simulink library "SpeakerSubsystemLibrary_1_0_0"  (R2022b)
settings: Solver=VariableStepAuto  StartTime=0.0  StopTime=10.0  RelTol=1e-3
undefined symbols (not defined in the file): BL_0, BL_1, BL_2, BL_3, BL_4, D_0, D_1, D_2, D_3, D_4, K_0, K_1, K_2, K_3, K_4, L2, Le_0, Le_1, Le_2, Le_3, Le_4, Mm, R2, Re, Sd
libraries: fl_lib x15, acoustical_lib x6
settings Model: Creator=stephenthompson  LastModifiedBy=sct12
settings ModelReferenceCC: EnableRefExpFcnMdlSchedulingChecks=on

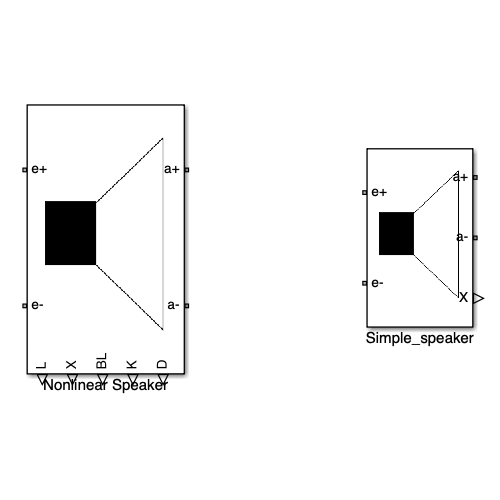
[thumbnail: Simulink's stored preview of the top-level diagram]
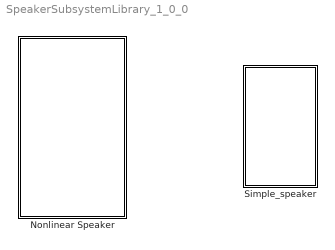
== system SpeakerSubsystemLibrary_1_0_0 ==
  Nonlinear Speaker : Subsystem  mask{Sd=Sd, Sd_unit=cm^2, Sd_conf=compiletime, mass=Mm, mass_unit=g, mass_conf=compiletime, R=Re, R_unit=Ohm, R_conf=compiletime, L2=L2, L2_unit=H, L2_conf=compiletime, R2=R2, R2_unit=Ohm, R2_conf=compiletime, L0_of_x=Le_0, L0_of_x_unit=H, L0_of_x_conf=compiletime, L1_of_x=Le_1, L1_of_x_unit=H/m, L1_of_x_conf=compiletime, L2_of_x=Le_2, L2_of_x_unit=H/m^2, L2_of_x_conf=compiletime, L3_of_x=Le_3, L3_of_x_unit=H/m^3, L3_of_x_conf=compiletime, L4_of_x=Le_4, L4_of_x_unit=H/m^4, L4_of_x_conf=compiletime, Bl0=BL_0, Bl0_unit=N/A, Bl0_conf=compiletime, Bl1=BL_1, Bl1_unit=N/(A*m), Bl1_conf=compiletime, Bl2=BL_2, Bl2_unit=N/(A*m^2), Bl2_conf=compiletime, Bl3=BL_3, Bl3_unit=N/(A*m^3), Bl3_conf=compiletime, Bl4=BL_4, Bl4_unit=N/(A*m^4), Bl4_conf=compiletime, K0=K_0, K0_unit=N/m, K0_conf=compiletime, K1=K_1, K1_unit=N/m^2, K1_conf=compiletime, K2=K_2, K2_unit=N/m^3, K2_conf=compiletime, K3=K_3, K3_unit=N/m^4, K3_conf=compiletime, K4=K_4, K4_unit=N/m^5, K4_conf=compiletime, D0=D_0, D0_unit=N*s/m, D0_conf=compiletime, D1=D_1, D1_unit=N*s^2/m^2, D1_conf=compiletime, D2=D_2, D2_unit=N*s^3/m^3, D2_conf=compiletime, D3=D_3, D3_unit=N*s^4/m^4, D3_conf=compiletime, D4=D_4, D4_unit=N*s^5/m^5, D4_conf=compiletime}
      mask prompts: Sd "Cone Area Sd"; mass "Moving Mass"; R "Coil Resistance"; Bl0 "Constant part in force factor"; Bl1 "1st order coefficient"; Bl2 "2nd order coefficient"; Bl3 "3rd order coefficient"; Bl4 "4th order coefficient"; K0 "constant part in stiffness"; K1 "1st order coefficient"; K2 "2nd order coefficient"; K3 "3rd order coefficient"; K4 "4th order coefficient"; D0 "constant part in stiffness"; D1 "N1st order coefficient"; D2 "N2nd order coefficient"; D3 "3rd order coefficient"; D4 "N*4th order coefficient"
      settings: PortSchema="{\"entries\":[{\"content\":{\"sides\":[{\"content\":{\"connectorIds\":[\"LConn1\",\"LConn2\"]},\"type\":\"ConnectorPlacement.EquallySpacedRectSide\",\"uuid\":\"f64a30bf-56c6-47b5-b4bc-71101fcbb95a\"},{\"content\":{\"connectorIds\":[\"RConn1\",\"RConn2\"],\"side\":\"RIGHT\"},\"type\":\"ConnectorPlacement.EquallySpacedRectSide\",\"uuid\":\"026264a5-a5ab-4ec3-912f-977c3d8fe047\"},{\"content\":{\"connectorIds\":[],\"side\":\"TOP\"},\"type\":\"ConnectorPlacement.EquallySpacedRectSide\",\"uuid\":\"73a10c58-d118-4274-a8f1-6138ac105e53\"},{\"content\":{\"connectorIds\":[\"RConn3\",\"RConn4\",\"RConn5\",\"RConn6\",\"RConn7\"],\"side\":\"BOTTOM\"},\"type\":\"ConnectorPlacement.EquallySpacedRectSide\",\"uuid\":\"493ec49a-e47d-475d-ab4f-1f36cc0e6d29\"}]},\"type\":\"ConnectorPlacement.EquallySpacedConnector\",\"uuid\":\"07e5b91c-fb95-4bee-828a-833440d87f91\"}],\"packageUris\":[\"http://schema.mathworks.com/mf0/Connector/R2020b\"],\"version\":\"1.0\"}"
      mask TypeOptions Sd: Area_xfrm/Sd
      mask TypeOptions Sd_unit: Area_xfrm/Sd_unit
      mask TypeOptions Sd_conf: Area_xfrm/Sd_conf
      mask TypeOptions mass: Mm/mass
      mask TypeOptions mass_unit: Mm/mass_unit
      mask TypeOptions mass_conf: Mm/mass_conf
      mask TypeOptions R: Re/R
      mask TypeOptions R_unit: Re/R_unit
      mask TypeOptions R_conf: Re/R_conf
      mask TypeOptions L2: L2/l
      mask TypeOptions L2_unit: L2/l_unit
      mask TypeOptions L2_conf: L2/l_conf
      mask TypeOptions R2: R2/R
      mask TypeOptions R2_unit: R2/R_unit
      mask TypeOptions R2_conf: R2/R_conf
      mask TypeOptions L0_of_x: Le_of_x/L0
      mask TypeOptions L0_of_x_unit: Le_of_x/L0_unit
      mask TypeOptions L0_of_x_conf: Le_of_x/L0_conf
      mask TypeOptions L1_of_x: Le_of_x/L1
      mask TypeOptions L1_of_x_unit: Le_of_x/L1_unit
      mask TypeOptions L1_of_x_conf: Le_of_x/L1_conf
      mask TypeOptions L2_of_x: Le_of_x/L2
      mask TypeOptions L2_of_x_unit: Le_of_x/L2_unit
      mask TypeOptions L2_of_x_conf: Le_of_x/L2_conf
      mask TypeOptions L3_of_x: Le_of_x/L3
      mask TypeOptions L3_of_x_unit: Le_of_x/L3_unit
      mask TypeOptions L3_of_x_conf: Le_of_x/L3_conf
      mask TypeOptions L4_of_x: Le_of_x/L4
      mask TypeOptions L4_of_x_unit: Le_of_x/L4_unit
      mask TypeOptions L4_of_x_conf: Le_of_x/L4_conf
      mask TypeOptions Bl0: BL_of_x/Bl0
      mask TypeOptions Bl0_unit: BL_of_x/Bl0_unit
      mask TypeOptions Bl0_conf: BL_of_x/Bl0_conf
      mask TypeOptions Bl1: BL_of_x/Bl1
      mask TypeOptions Bl1_unit: BL_of_x/Bl1_unit
      mask TypeOptions Bl1_conf: BL_of_x/Bl1_conf
      mask TypeOptions Bl2: BL_of_x/Bl2
      mask TypeOptions Bl2_unit: BL_of_x/Bl2_unit
      mask TypeOptions Bl2_conf: BL_of_x/Bl2_conf
      mask TypeOptions Bl3: BL_of_x/Bl3
      mask TypeOptions Bl3_unit: BL_of_x/Bl3_unit
      mask TypeOptions Bl3_conf: BL_of_x/Bl3_conf
      mask TypeOptions Bl4: BL_of_x/Bl4
      mask TypeOptions Bl4_unit: BL_of_x/Bl4_unit
      mask TypeOptions Bl4_conf: BL_of_x/Bl4_conf
      mask TypeOptions K0: K_of_x/K0
      mask TypeOptions K0_unit: K_of_x/K0_unit
      mask TypeOptions K0_conf: K_of_x/K0_conf
      mask TypeOptions K1: K_of_x/K1
      mask TypeOptions K1_unit: K_of_x/K1_unit
      mask TypeOptions K1_conf: K_of_x/K1_conf
      mask TypeOptions K2: K_of_x/K2
      mask TypeOptions K2_unit: K_of_x/K2_unit
      mask TypeOptions K2_conf: K_of_x/K2_conf
      mask TypeOptions K3: K_of_x/K3
      mask TypeOptions K3_unit: K_of_x/K3_unit
      mask TypeOptions K3_conf: K_of_x/K3_conf
      mask TypeOptions K4: K_of_x/K4
      mask TypeOptions K4_unit: K_of_x/K4_unit
      mask TypeOptions K4_conf: K_of_x/K4_conf
      mask TypeOptions D0: Rm_of_v/D0
      mask TypeOptions D0_unit: Rm_of_v/D0_unit
      mask TypeOptions D0_conf: Rm_of_v/D0_conf
      mask TypeOptions D1: Rm_of_v/D1
      mask TypeOptions D1_unit: Rm_of_v/D1_unit
      mask TypeOptions D1_conf: Rm_of_v/D1_conf
      mask TypeOptions D2: Rm_of_v/D2
      mask TypeOptions D2_unit: Rm_of_v/D2_unit
      mask TypeOptions D2_conf: Rm_of_v/D2_conf
      mask TypeOptions D3: Rm_of_v/D3
      mask TypeOptions D3_unit: Rm_of_v/D3_unit
      mask TypeOptions D3_conf: Rm_of_v/D3_conf
      mask TypeOptions D4: Rm_of_v/D4
      mask TypeOptions D4_unit: Rm_of_v/D4_unit
      mask TypeOptions D4_conf: Rm_of_v/D4_conf
      mask DialogControl Container4 Prompt: Inductor Parameters
      mask DialogControl Container5 Prompt: Force Factor BL Parameters
      mask DialogControl Container6 Prompt: Spring Stiffness Parameters
      mask DialogControl Container7 Prompt: Mechanical Damping Parameters
      mask Display: image('$imagefile'); % Use "Edit Image" on toolstrip to change.
  Simple_speaker : Subsystem  mask{Re=7.8, Re_unit=Ohm, Re_conf=compiletime, Le=0.124, Le_unit=H, Le_conf=compiletime, L2=1e-6, L2_unit=H, L2_conf=compiletime, R2=1, R2_unit=Ohm, R2_conf=compiletime, BL=5.63, BL_unit=V*s/m, BL_conf=compiletime, Mm=4.8, Mm_unit=g, Mm_conf=compiletime, K=1/1.05e-3, K_unit=N/m, K_conf=compiletime, D=1, D_unit=N*s/m, D_conf=compiletime, Sd=30.4, Sd_unit=cm^2, Sd_conf=compiletime}
      mask prompts: Re "Coil Resistance"; Le "Coil Inductance"; BL "Force Factor BL"; Mm "Cone Moving Mass"; K "Cone Mounting Stiffness"; D "Mechanical Resistance"; Sd "Cone Area"
      mask TypeOptions Re: Re/R
      mask TypeOptions Re_unit: Re/R_unit
      mask TypeOptions Re_conf: Re/R_conf
      mask TypeOptions Le: Le/l
      mask TypeOptions Le_unit: Le/l_unit
      mask TypeOptions Le_conf: Le/l_conf
      mask TypeOptions L2: L2/l
      mask TypeOptions L2_unit: L2/l_unit
      mask TypeOptions L2_conf: L2/l_conf
      mask TypeOptions R2: R2/R
      mask TypeOptions R2_unit: R2/R_unit
      mask TypeOptions R2_conf: R2/R_conf
      mask TypeOptions BL: BL/K
      mask TypeOptions BL_unit: BL/K_unit
      mask TypeOptions BL_conf: BL/K_conf
      mask TypeOptions Mm: Mm/mass
      mask TypeOptions Mm_unit: Mm/mass_unit
      mask TypeOptions Mm_conf: Mm/mass_conf
      mask TypeOptions K: K/spr_rate
      mask TypeOptions K_unit: K/spr_rate_unit
      mask TypeOptions K_conf: K/spr_rate_conf
      mask TypeOptions D: D/D
      mask TypeOptions D_unit: D/D_unit
      mask TypeOptions D_conf: D/D_conf
      mask TypeOptions Sd: Sd/Sd
      mask TypeOptions Sd_unit: Sd/Sd_unit
      mask TypeOptions Sd_conf: Sd/Sd_conf
      mask Display: image('$imagefile'); % Use "Edit Image" on toolstrip to change.

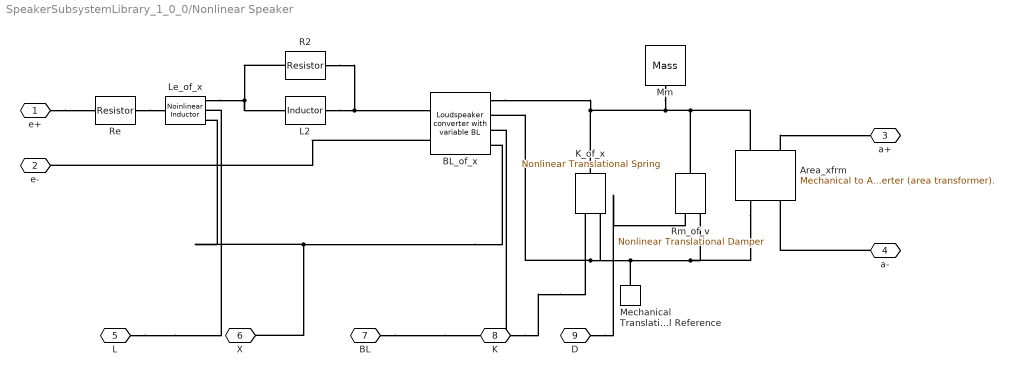
== system SpeakerSubsystemLibrary_1_0_0/Nonlinear Speaker ==
  Area_xfrm : acoustical_lib/Acoustical Elements/Mechanical to Acoustical Converter (area transformer).  Sd=Sd cm^2  u_specify=off  u_priority=None  u=0 m^3/s  u_nominal_specify=off  u_nominal_unit=m^3/s  u_nominal_value=1  p_specify=off  p_priority=None  p=0 Pa  p_nominal_specify=off  p_nominal_unit=Pa  p_nominal_value=1  f_specify=off  f_priority=None  f=0 N  f_nominal_specify=off  f_nominal_unit=N  f_nominal_value=1  v_specify=off  v_priority=None  v=0 m/s  v_nominal_specify=off  v_nominal_unit=m/s  v_nominal_value=1
      settings: SourceProductName=Acoustical  InternalSimscapePortConfiguration="{\"Bottom\":[],\"Left\":[{\"id\":\"pp\",\"label\":\"+\",\"type\":\"acoustical.acoustical\"},{\"id\":\"R\",\"label\":\"R\",\"type\":\"foundation.mechanical.translational.translational\"}],\"Right\":[{\"id\":\"nn\",\"label\":\"-\",\"type\":\"acoustical.acoustical\"},{\"id\":\"C\",\"label\":\"C\",\"type\":\"foundation.mechanical.translational.translational\"}],\"Top\":[]}"
  BL_of_x : acoustical_lib/Moving Coil Speakers/speaker_nonlinear_blocks/Loudspeaker converter with variable BL  Bl0=Bl0 N/A  Bl1=Bl1 N/(A*m)  Bl2=Bl2 N/(A*m^2)  Bl3=Bl3 N/(A*m^3)  Bl4=Bl4 N/(A*m^4)  i_specify=off  i_priority=None  i=0 A  i_nominal_specify=off  i_nominal_unit=A  i_nominal_value=1  v_specify=off  v_priority=None  v=0 V  v_nominal_specify=off  v_nominal_unit=V  v_nominal_value=1  f_specify=off  f_priority=None  f=0 N  f_nominal_specify=off  f_nominal_unit=N  f_nominal_value=1  u_specify=off  u_priority=None  u=0 m/s  u_nominal_specify=off  u_nominal_unit=m/s  u_nominal_value=1
      settings: SourceProductName=Acoustical  InternalSimscapePortConfiguration="{\"Bottom\":[{\"id\":\"BL\",\"label\":\"BL\",\"type\":\"output\"},{\"id\":\"X\",\"label\":\"\",\"type\":\"output\"}],\"Left\":[{\"id\":\"p\",\"label\":\"+\",\"type\":\"foundation.electrical.electrical\"},{\"id\":\"n\",\"label\":\"-\",\"type\":\"foundation.electrical.electrical\"}],\"Right\":[{\"id\":\"R\",\"label\":\"R\",\"type\":\"foundation.mechanical.translational.translational\"},{\"id\":\"C\",\"label\":\"C\",\"type\":\"foundation.mechanical.translational.translational\"}],\"Top\":[]}"
  K_of_x : acoustical_lib/Moving Coil Speakers/speaker_nonlinear_blocks/Nonlinear Translational Spring  K0=K0 N/m  K1=K1 N/m^2  K2=K2 N/m^3  K3=K3 N/m^4  K4=K4 N/m^5  v_specify=off  v_priority=None  v=0 m/s  v_nominal_specify=off  v_nominal_unit=m/s  v_nominal_value=1  f_specify=off  f_priority=None  f=0 N  f_nominal_specify=off  f_nominal_unit=N  f_nominal_value=1  x_specify=off  x_priority=High  x=0 m  x_nominal_specify=off  x_nominal_unit=m  x_nominal_value=1
      settings: SourceProductName=Acoustical  InternalSimscapePortConfiguration="{\"Bottom\":[{\"id\":\"K\",\"label\":\"K\",\"type\":\"output\"}],\"Left\":[{\"id\":\"R\",\"label\":\"R\",\"type\":\"foundation.mechanical.translational.translational\"}],\"Right\":[{\"id\":\"C\",\"label\":\"C\",\"type\":\"foundation.mechanical.translational.translational\"}],\"Top\":[]}"
  L2 : fl_lib/Electrical/Electrical Elements/Inductor  l=L2 H  r=0 Ohm  g=1e-9 1/Ohm  i_specify=off  i_priority=None  i=0 A  i_nominal_specify=off  i_nominal_unit=A  i_nominal_value=1  v_specify=off  v_priority=None  v=0 V  v_nominal_specify=off  v_nominal_unit=V  v_nominal_value=1  i_L_specify=off  i_L_priority=High  i_L=0 A  i_L_nominal_specify=off  i_L_nominal_unit=A  i_L_nominal_value=1
  Le_of_x : acoustical_lib/Moving Coil Speakers/speaker_nonlinear_blocks/Noinlinear Inductor  r=0 Ohm  g=1e-9 1/Ohm  L0=L0_of_x H  L1=L1_of_x H/m  L2=L2_of_x H/m^2  L3=L3_of_x H/m^3  L4=L4_of_x H/m^4  i_specify=off  i_priority=None  i=0 A  i_nominal_specify=off  i_nominal_unit=A  i_nominal_value=1  v_specify=off  v_priority=None  v=0 V  v_nominal_specify=off  v_nominal_unit=V  v_nominal_value=1  i_L_specify=off  i_L_priority=High  i_L=0 A  i_L_nominal_specify=off  i_L_nominal_unit=A  i_L_nominal_value=1
      settings: SourceProductName=Acoustical  InternalSimscapePortConfiguration="{\"Bottom\":[{\"id\":\"L\",\"label\":\"L\",\"type\":\"output\"},{\"id\":\"X\",\"label\":\"x\",\"type\":\"input\"}],\"Left\":[{\"id\":\"p\",\"label\":\"+\",\"type\":\"foundation.electrical.electrical\"}],\"Right\":[{\"id\":\"n\",\"label\":\"-\",\"type\":\"foundation.electrical.electrical\"}],\"Top\":[]}"
  Mechanical Translational Reference : fl_lib/Mechanical/Translational Elements/Mechanical Translational Reference
  Mm : fl_lib/Mechanical/Translational Elements/Mass  mass=mass g  num_ports=foundation.enum.numPorts2.one  v_specify=off  v_priority=High  v=0 m/s  v_nominal_specify=off  v_nominal_unit=m/s  v_nominal_value=1  f_specify=off  f_priority=None  f=0 N  f_nominal_specify=off  f_nominal_unit=N  f_nominal_value=1
  R2 : fl_lib/Electrical/Electrical Elements/Resistor  R=R2 Ohm  i_specify=off  i_priority=None  i=0 A  i_nominal_specify=off  i_nominal_unit=A  i_nominal_value=1  v_specify=off  v_priority=None  v=0 V  v_nominal_specify=off  v_nominal_unit=V  v_nominal_value=1
  Re : fl_lib/Electrical/Electrical Elements/Resistor  R=R Ohm  i_specify=off  i_priority=None  i=0 A  i_nominal_specify=off  i_nominal_unit=A  i_nominal_value=1  v_specify=off  v_priority=None  v=0 V  v_nominal_specify=off  v_nominal_unit=V  v_nominal_value=1
  Rm_of_v : acoustical_lib/Moving Coil Speakers/speaker_nonlinear_blocks/Nonlinear Translational Damper  D0=D0 N*s/m  D1=D1 N*s^2/m^2  D2=D2 N*s^3/m^3  D3=D3 N*s^4/m^4  D4=D4 N*s^5/m^5  v_specify=off  v_priority=None  v=0 m/s  v_nominal_specify=off  v_nominal_unit=m/s  v_nominal_value=1  f_specify=off  f_priority=None  f=0 N  f_nominal_specify=off  f_nominal_unit=N  f_nominal_value=1  x_specify=off  x_priority=High  x=0 m  x_nominal_specify=off  x_nominal_unit=m  x_nominal_value=1
      settings: SourceProductName=Acoustical  InternalSimscapePortConfiguration="{\"Bottom\":[{\"id\":\"D\",\"label\":\"D\",\"type\":\"output\"}],\"Left\":[{\"id\":\"R\",\"label\":\"R\",\"type\":\"foundation.mechanical.translational.translational\"}],\"Right\":[{\"id\":\"C\",\"label\":\"C\",\"type\":\"foundation.mechanical.translational.translational\"}],\"Top\":[]}"
  e+ : PMIOPort  Side=Left
  e- : PMIOPort  Port=2  Side=Left
  a+ : PMIOPort  Port=3  Side=Right
  a- : PMIOPort  Port=4  Side=Right
  L : PMIOPort  Port=5  Side=Right
  X : PMIOPort  Port=6  Side=Right
  BL : PMIOPort  Port=7  Side=Right
  K : PMIOPort  Port=8  Side=Right
  D : PMIOPort  Port=9  Side=Right
  connections:
  X/RConn1 -- BL_of_x/RConn4 -- Le_of_x/RConn3
  e+/RConn1 -- Re/LConn1
  Rm_of_v/LConn1 -- Area_xfrm/LConn2 -- Mm/LConn1 -- K_of_x/LConn1 -- BL_of_x/RConn1
  Re/RConn1 -- Le_of_x/LConn1
  Area_xfrm/LConn1 -- a+/RConn1
  D/RConn1 -- Rm_of_v/RConn2
  BL_of_x/LConn2 -- e-/RConn1
  Area_xfrm/RConn2 -- Mechanical Translational Reference/LConn1 -- BL_of_x/RConn2 -- K_of_x/RConn1 -- Rm_of_v/RConn1
  L/RConn1 -- Le_of_x/RConn2
  BL/RConn1 -- BL_of_x/RConn3
  K/RConn1 -- K_of_x/RConn2
  a-/RConn1 -- Area_xfrm/RConn1
  Le_of_x/RConn1 -- R2/LConn1 -- L2/LConn1
  L2/RConn1 -- R2/RConn1 -- BL_of_x/LConn1

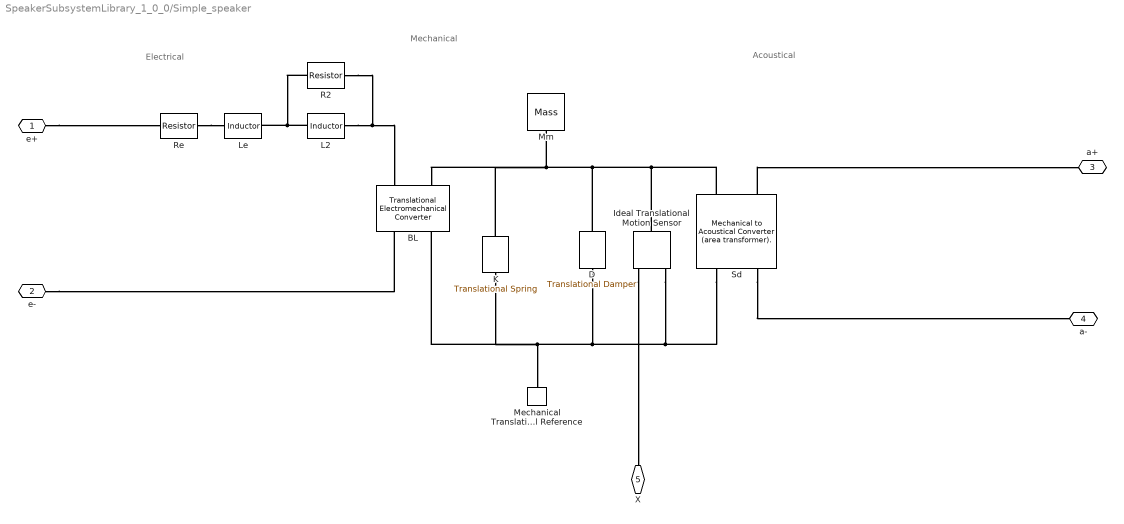
== system SpeakerSubsystemLibrary_1_0_0/Simple_speaker ==
  note: Acoustical
  note: Mechanical
  note: Electrical
  BL : fl_lib/Electrical/Electrical Elements/Translational Electromechanical Converter  K=BL V*s/m  i_specify=off  i_priority=None  i=0 A  i_nominal_specify=off  i_nominal_unit=A  i_nominal_value=1  v_specify=off  v_priority=None  v=0 V  v_nominal_specify=off  v_nominal_unit=V  v_nominal_value=1  f_specify=off  f_priority=None  f=0 N  f_nominal_specify=off  f_nominal_unit=N  f_nominal_value=1  u_specify=off  u_priority=None  u=0 m/s  u_nominal_specify=off  u_nominal_unit=m/s  u_nominal_value=1
      settings: InternalSimscapePortConfiguration="{\"Bottom\":[],\"Left\":[{\"id\":\"p\",\"label\":\"+\",\"type\":\"foundation.electrical.electrical\"},{\"id\":\"R\",\"label\":\"R\",\"type\":\"foundation.mechanical.translational.translational\"}],\"Right\":[{\"id\":\"n\",\"label\":\"-\",\"type\":\"foundation.electrical.electrical\"},{\"id\":\"C\",\"label\":\"C\",\"type\":\"foundation.mechanical.translational.translational\"}],\"Top\":[]}"
  D : fl_lib/Mechanical/Translational Elements/Translational Damper  D=D N*s/m  v_specify=off  v_priority=None  v=0 m/s  v_nominal_specify=off  v_nominal_unit=m/s  v_nominal_value=1  f_specify=off  f_priority=None  f=0 N  f_nominal_specify=off  f_nominal_unit=N  f_nominal_value=1
  Ideal Translational Motion Sensor : fl_lib/Mechanical/Mechanical Sensors/Ideal Translational Motion Sensor  reference=foundation.enum.MeasurementReference.difference  acceleration_port=false  velocity_port=true  position_port=true  offset=0 m
  K : fl_lib/Mechanical/Translational Elements/Translational Spring  spr_rate=K N/m  v_specify=off  v_priority=None  v=0 m/s  v_nominal_specify=off  v_nominal_unit=m/s  v_nominal_value=1  f_specify=off  f_priority=None  f=0 N  f_nominal_specify=off  f_nominal_unit=N  f_nominal_value=1  x_specify=off  x_priority=High  x=0 m  x_nominal_specify=off  x_nominal_unit=m  x_nominal_value=1
  L2 : fl_lib/Electrical/Electrical Elements/Inductor  l=L2 H  r=0 Ohm  g=1e-9 1/Ohm  i_specify=off  i_priority=None  i=0 A  i_nominal_specify=off  i_nominal_unit=A  i_nominal_value=1  v_specify=off  v_priority=None  v=0 V  v_nominal_specify=off  v_nominal_unit=V  v_nominal_value=1  i_L_specify=off  i_L_priority=High  i_L=0 A  i_L_nominal_specify=off  i_L_nominal_unit=A  i_L_nominal_value=1
  Le : fl_lib/Electrical/Electrical Elements/Inductor  l=Le H  r=0 Ohm  g=1e-9 1/Ohm  i_specify=off  i_priority=None  i=0 A  i_nominal_specify=off  i_nominal_unit=A  i_nominal_value=1  v_specify=off  v_priority=None  v=0 V  v_nominal_specify=off  v_nominal_unit=V  v_nominal_value=1  i_L_specify=off  i_L_priority=High  i_L=0 A  i_L_nominal_specify=off  i_L_nominal_unit=A  i_L_nominal_value=1
  Mechanical Translational Reference : fl_lib/Mechanical/Translational Elements/Mechanical Translational Reference
  Mm : fl_lib/Mechanical/Translational Elements/Mass  mass=Mm g  num_ports=foundation.enum.numPorts2.one  v_specify=off  v_priority=High  v=0 m/s  v_nominal_specify=off  v_nominal_unit=m/s  v_nominal_value=1  f_specify=off  f_priority=None  f=0 N  f_nominal_specify=off  f_nominal_unit=N  f_nominal_value=1
  R2 : fl_lib/Electrical/Electrical Elements/Resistor  R=R2 Ohm  i_specify=off  i_priority=None  i=0 A  i_nominal_specify=off  i_nominal_unit=A  i_nominal_value=1  v_specify=off  v_priority=None  v=0 V  v_nominal_specify=off  v_nominal_unit=V  v_nominal_value=1
  Re : fl_lib/Electrical/Electrical Elements/Resistor  R=Re Ohm  i_specify=off  i_priority=None  i=0 A  i_nominal_specify=off  i_nominal_unit=A  i_nominal_value=1  v_specify=off  v_priority=None  v=0 V  v_nominal_specify=off  v_nominal_unit=V  v_nominal_value=1
  Sd : acoustical_lib/Acoustical Elements/Mechanical to Acoustical Converter (area transformer).  Sd=Sd cm^2  u_specify=off  u_priority=None  u=0 m^3/s  u_nominal_specify=off  u_nominal_unit=m^3/s  u_nominal_value=1  p_specify=off  p_priority=None  p=0 Pa  p_nominal_specify=off  p_nominal_unit=Pa  p_nominal_value=1  f_specify=off  f_priority=None  f=0 N  f_nominal_specify=off  f_nominal_unit=N  f_nominal_value=1  v_specify=off  v_priority=None  v=0 m/s  v_nominal_specify=off  v_nominal_unit=m/s  v_nominal_value=1
      settings: SourceProductName=Acoustical  InternalSimscapePortConfiguration="{\"Bottom\":[],\"Left\":[{\"id\":\"pp\",\"label\":\"+\",\"type\":\"acoustical.acoustical\"},{\"id\":\"R\",\"label\":\"R\",\"type\":\"foundation.mechanical.translational.translational\"}],\"Right\":[{\"id\":\"nn\",\"label\":\"-\",\"type\":\"acoustical.acoustical\"},{\"id\":\"C\",\"label\":\"C\",\"type\":\"foundation.mechanical.translational.translational\"}],\"Top\":[]}"
  e+ : PMIOPort  Side=Left
  e- : PMIOPort  Port=2  Side=Left
  a+ : PMIOPort  Port=3  Side=Right
  a- : PMIOPort  Port=4  Side=Right
  X : PMIOPort  Port=5  Side=Right
  connections:
  e-/RConn1 -- BL/RConn1
  Sd/LConn1 -- a+/RConn1
  e+/RConn1 -- Re/LConn1
  Sd/RConn2 -- Ideal Translational Motion Sensor/RConn1 -- D/RConn1 -- K/RConn1 -- BL/RConn2 -- Mechanical Translational Reference/LConn1
  Sd/RConn1 -- a-/RConn1
  Sd/LConn2 -- Ideal Translational Motion Sensor/LConn1 -- D/LConn1 -- K/LConn1 -- BL/LConn2 -- Mm/LConn1
  Re/RConn1 -- Le/LConn1
  L2/LConn1 -- R2/LConn1 -- Le/RConn1
  L2/RConn1 -- R2/RConn1 -- BL/LConn1
  Ideal Translational Motion Sensor/RConn3 -- X/RConn1
